simulink model "Model21"  (R2020a)
settings: Solver=VariableStepAuto  StartTime=0.0  StopTime=10.0  RelTol=1e-3
settings Model: Creator=HP  LastModifiedBy=HP

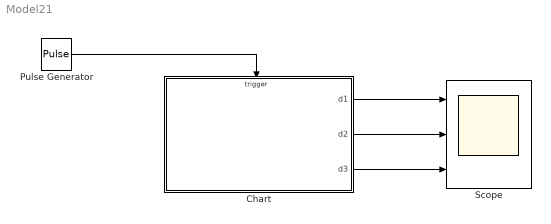
== system Model21 ==
  Chart : Stateflow chart  TreatAsAtomicUnit=on
  Pulse Generator : DiscretePulseGenerator  PulseType=Time based  Period=0.1  PulseWidth=5
  Scope : Scope  NumInputPorts=3
  wires:
  Chart/1(d1) -> Scope/1
  Chart/2(d2) -> Scope/2
  Pulse Generator/1 -> Chart/Trigger
  Chart/3(d3) -> Scope/3

== stateflow chart Model21/Chart ==
  state DigitTwo [parallel]
    settings: executionOrder=2
    state One
      en:
      d2=1;
    state Two
      en:
      d2=2;
    state Zero
      en:
      d2=0;
    state Four
      en:
      d2=4;
    state Three
      en:
      d2=3;
    DigitTwo.One -> DigitTwo.Two : SecondClick
    DigitTwo.Zero -> DigitTwo.One : SecondClick
    DigitTwo.Two -> DigitTwo.Three : SecondClick
    (default) -> DigitTwo.Zero
    DigitTwo.Four -> DigitTwo.Zero : SecondClick/{ThirdClick}
    DigitTwo.Three -> DigitTwo.Four : SecondClick
  state DigitOne [parallel]
    settings: executionOrder=1
    state One
      en:
      d1=1;
    state Two
      en:
      d1=2;
    state Zero
      en:
      d1=0;
    state Four
      en:
      d1=4;
    state Three
      en:
      d1=3;
    DigitOne.One -> DigitOne.Two : FirstClick
    DigitOne.Zero -> DigitOne.One : FirstClick
    DigitOne.Two -> DigitOne.Three : FirstClick
    (default) -> DigitOne.Zero
    DigitOne.Four -> DigitOne.Zero : FirstClick/{SecondClick}
    DigitOne.Three -> DigitOne.Four : FirstClick
  state DigitThree [parallel]
    settings: executionOrder=3
    state One
      en:
      d3=1;
    state Two
      en:
      d3=2;
    state Zero
      en:
      d3=0;
    state Four
      en:
      d3=4;
    state Three
      en:
      d3=3;
    DigitThree.One -> DigitThree.Two : ThirdClick
    DigitThree.Zero -> DigitThree.One : ThirdClick
    DigitThree.Two -> DigitThree.Three : ThirdClick
    (default) -> DigitThree.Zero
    DigitThree.Four -> DigitThree.Zero : ThirdClick
    DigitThree.Three -> DigitThree.Four : ThirdClick
  (default) -> DigitOne
  data: d1 output; d2 output; d3 output
  events: FirstClick input RISING_EDGE_EVENT; SecondClick local FUNCTION_CALL_EVENT; ThirdClick local FUNCTION_CALL_EVENT
